simulink model "lqrsim"  (R2024b)
settings: Solver=VariableStepAuto  StartTime=0.0  StopTime=20  RelTol=1e-3
undefined symbols (not defined in the file or in its folder): dirsorder, dtflin, lqrtflin, PpReg
settings Model: Creator=markminerov  LastModifiedBy=markminerov
settings DebuggingCC: AlgebraicLoopMsg=none

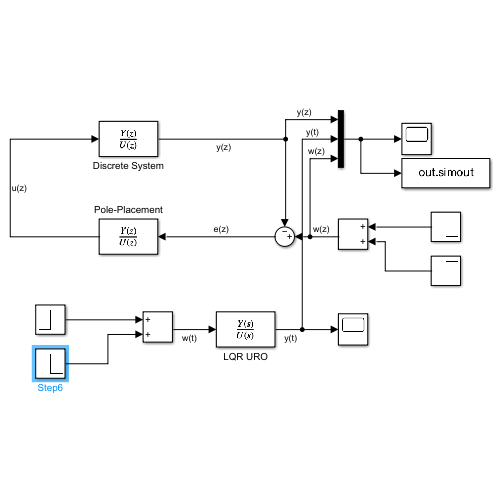
[thumbnail: Simulink's stored preview of the top-level diagram]
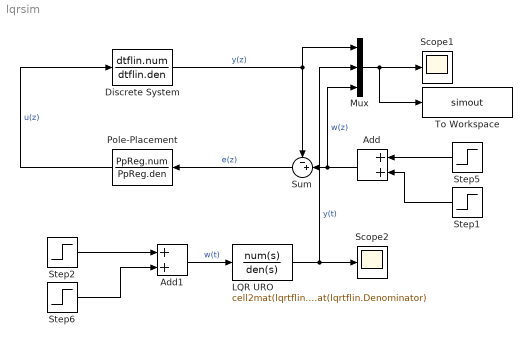
== system lqrsim ==
  Add : Sum
  Add1 : Sum
  Discrete System : DiscreteTransferFcn  Numerator=dtflin.num  Denominator=dtflin.den
  LQR URO : TransferFcn  Numerator=cell2mat(lqrtflin.Numerator)  Denominator=cell2mat(lqrtflin.Denominator)
  Mux : Mux  Inputs=3
  Pole-Placement : DiscreteTransferFcn  Numerator=PpReg.num  Denominator=PpReg.den
  Scope1 : Scope
  Scope2 : Scope
  Step1 : Step  SampleTime=0
  Step2 : Step  SampleTime=0
  Step5 : Step  Time=dirsorder(1)  After=-1  SampleTime=0
  Step6 : Step  Time=dirsorder(1)  After=-1  SampleTime=0
  Sum : Sum  Inputs=-+|
  To Workspace : ToWorkspace  VariableName=simout  SaveFormat=Timeseries  SampleTime=-1
  wires:
  Add/1 -> Mux/3, Sum/2  "w(z)"
  Sum/1 -> Pole-Placement/1  "e(z)"
  Pole-Placement/1 -> Discrete System/1  "u(z)"
  Mux/1 -> To Workspace/1, Scope1/1
  Discrete System/1 -> Mux/1, Sum/1  "y(z)"
  Step2/1 -> Add1/1
  Step6/1 -> Add1/2
  LQR URO/1 -> Mux/2, Scope2/1  "y(t)"
  Add1/1 -> LQR URO/1  "w(t)"
  Step5/1 -> Add/1
  Step1/1 -> Add/2
